simulink model "AOO"  (R2020a)
settings: Solver=FixedStepAuto  StartTime=0.0  StopTime=10.0  FixedStep=1e-3  RelTol=1e-3  EnableMultiTasking=on
undefined symbols (not defined in the file): D10, D11, D12, D2, D4, D5, D7, D8, D9, PTA0, PTA2, PTB23, PTB9, PTC3, PTC4, PTD0, PTD2, PTD3
libraries: frdmk64flib x11
settings Model: ExtModeTrigDuration=5  Creator=Hasan  LastModifiedBy=Hasan
settings OptimizationCC: EnhancedBackFolding=on  PassReuseOutputArgsAs=Individual arguments  ZeroExternalMemoryAtStartup=off  ZeroInternalMemoryAtStartup=off  MaxStackSize=64  OptimizeBlockOrder=speed  DifferentSizesBufferReuse=on  OptimizationCustomize=off  EfficientTunableParamExpr=on
settings DebuggingCC: ParameterTunabilityLossMsg=error
settings HardwareCC: ProdBitPerPointer=32  ProdBitPerSizeT=32  ProdBitPerPtrDiffT=32  ProdLargestAtomicInteger=Long  ProdLargestAtomicFloat=Double  ProdWordSize=32  ProdHWDeviceType=ARM Compatible->ARM Cortex
settings SFSimCC: MATLABDynamicMemAlloc=off
settings RTWCC: SystemTargetFile=ert.tlc  HardwareBoard=NXP FRDM-K64F  TemplateMakefile=ert_default_tmf  Toolchain=GNU Tools for ARM Embedded Processors
settings CodeAppCC: ForceParamTrailComments=on  IgnoreCustomStorageClasses=off  OperatorAnnotations=on  SimulinkDataObjDesc=on  SFDataObjDesc=on  InsertBlockDesc=on

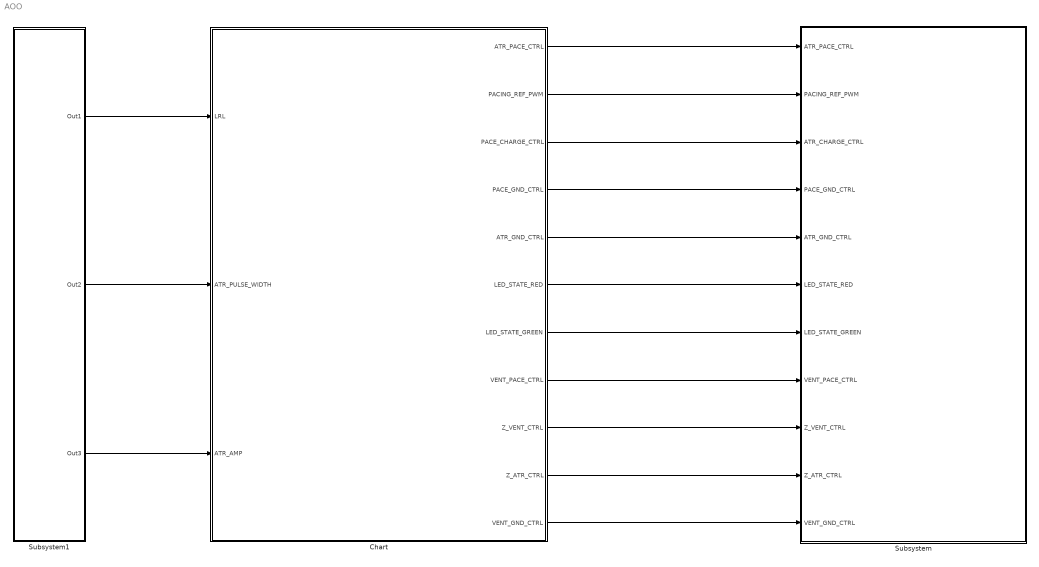
== system AOO ==
  Chart : Stateflow chart  TreatAsAtomicUnit=on
  Subsystem : Subsystem
  Subsystem1 : Subsystem
  wires:
  Chart/4(PACE_GND_CTRL) -> Subsystem/4(PACE_GND_CTRL)
  Chart/5(ATR_GND_CTRL) -> Subsystem/5(ATR_GND_CTRL)
  Chart/10(Z_ATR_CTRL) -> Subsystem/10(Z_ATR_CTRL)
  Chart/2(PACING_REF_PWM) -> Subsystem/2(PACING_REF_PWM)
  Chart/6(LED_STATE_RED) -> Subsystem/6(LED_STATE_RED)
  Chart/7(LED_STATE_GREEN) -> Subsystem/7(LED_STATE_GREEN)
  Chart/9(Z_VENT_CTRL) -> Subsystem/9(Z_VENT_CTRL)
  Chart/11(VENT_GND_CTRL) -> Subsystem/11(VENT_GND_CTRL)
  Chart/8(VENT_PACE_CTRL) -> Subsystem/8(VENT_PACE_CTRL)
  Chart/1(ATR_PACE_CTRL) -> Subsystem/1(ATR_PACE_CTRL)
  Chart/3(PACE_CHARGE_CTRL) -> Subsystem/3(ATR_CHARGE_CTRL)
  Subsystem1/1(Out1) -> Chart/1(LRL)
  Subsystem1/2(Out2) -> Chart/2(ATR_PULSE_WIDTH)
  Subsystem1/3(Out3) -> Chart/3(ATR_AMP)

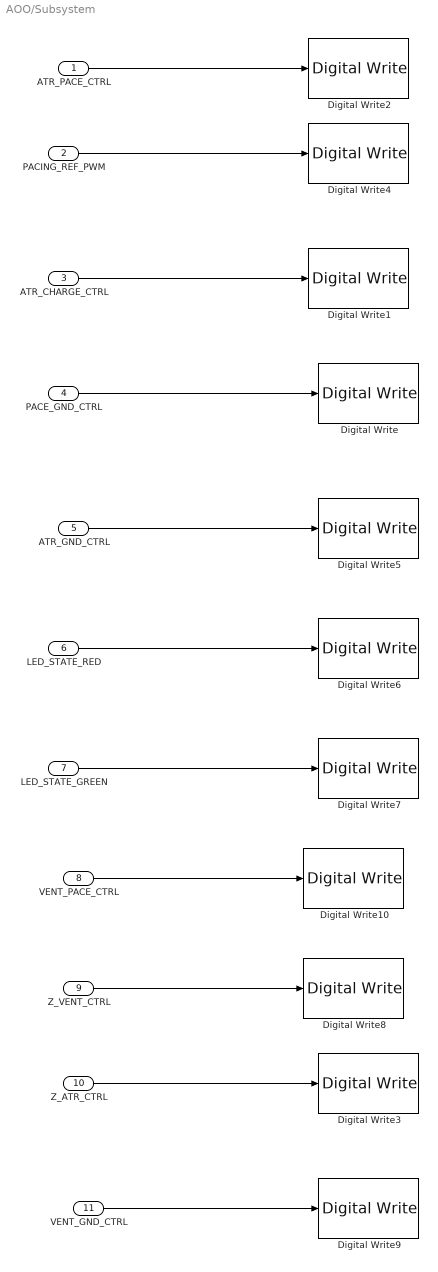
== system AOO/Subsystem ==
  ATR_PACE_CTRL : Inport
  PACING_REF_PWM : Inport  Port=2
  ATR_CHARGE_CTRL : Inport  Port=3
  PACE_GND_CTRL : Inport  Port=4
  ATR_GND_CTRL : Inport  Port=5
  LED_STATE_RED : Inport  Port=6
  LED_STATE_GREEN : Inport  Port=7
  VENT_PACE_CTRL : Inport  Port=8
  Z_VENT_CTRL : Inport  Port=9
  Z_ATR_CTRL : Inport  Port=10
  VENT_GND_CTRL : Inport  Port=11
  Digital Write : frdmk64flib/Digital Write  Whichpin=PTD0 (D10)
  Digital Write1 : frdmk64flib/Digital Write  Whichpin=PTB9 (D2)
  Digital Write10 : frdmk64flib/Digital Write  Whichpin=PTC4 (D9)
  Digital Write2 : frdmk64flib/Digital Write  Whichpin=PTA0 (D8)
  Digital Write3 : frdmk64flib/Digital Write  Whichpin=PTB23 (D4)
  Digital Write4 : frdmk64flib/Digital Write  Whichpin=PTA2 (D5)
  Digital Write5 : frdmk64flib/Digital Write  Whichpin=PTD2 (D11)
  Digital Write6 : frdmk64flib/Digital Write  Whichpin=RED_LED
  Digital Write7 : frdmk64flib/Digital Write  Whichpin=GREEN_LED
  Digital Write8 : frdmk64flib/Digital Write  Whichpin=PTC3 (D7)
  Digital Write9 : frdmk64flib/Digital Write  Whichpin=PTD3 (D12)
  wires:
  ATR_PACE_CTRL/1 -> Digital Write2/1
  PACING_REF_PWM/1 -> Digital Write4/1
  ATR_CHARGE_CTRL/1 -> Digital Write1/1
  VENT_GND_CTRL/1 -> Digital Write9/1
  Z_ATR_CTRL/1 -> Digital Write3/1
  Z_VENT_CTRL/1 -> Digital Write8/1
  VENT_PACE_CTRL/1 -> Digital Write10/1
  LED_STATE_GREEN/1 -> Digital Write7/1
  LED_STATE_RED/1 -> Digital Write6/1
  ATR_GND_CTRL/1 -> Digital Write5/1
  PACE_GND_CTRL/1 -> Digital Write/1

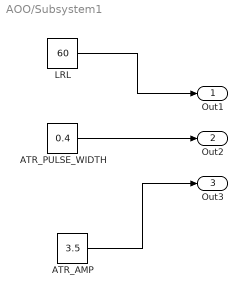
== system AOO/Subsystem1 ==
  ATR_AMP : Constant  Value=3.5  OutDataTypeStr=double
  ATR_PULSE_WIDTH : Constant  Value=0.4  OutDataTypeStr=double
  LRL : Constant  Value=60  OutDataTypeStr=double
  Out1 : Outport
  Out2 : Outport  Port=2
  Out3 : Outport  Port=3
  wires:
  ATR_AMP/1 -> Out3/1
  ATR_PULSE_WIDTH/1 -> Out2/1
  LRL/1 -> Out1/1

== stateflow chart AOO/Chart ==
  state AOO_INTERVAL_TIMER
    entry:
    ATR_PACE_CTRL = 0;
    PACE_CHARGE_CTRL = 1;
    PACING_REF_PWM = ATR_AMP;
    ATR_GND_CTRL = 1;
    PACE_GND_CTRL = 1;
    VENT_PACE_CTRL = 0;
    VENT_GND_CTRL = 0;
    Z_ATR_CTRL = 0;
    LED_STATE_RED=true;
    LED_STATE_GREEN=false;
  state AOO_PACE_DELIVERY
    entry:
    ATR_PACE_CTRL = 1;
    PACE_CHARGE_CTRL = 0;
    ATR_GND_CTRL = 0;
    PACE_GND_CTRL = 1;
    VENT_PACE_CTRL = 0;
    VENT_GND_CTRL = 0;
    Z_VENT_CTRL = 0;
    LED_STATE_RED=false;
    LED_STATE_GREEN=true;
  AOO_INTERVAL_TIMER -> AOO_PACE_DELIVERY : [after(60000/LRL-ATR_PULSE_WIDTH,msec)]
  AOO_PACE_DELIVERY -> AOO_INTERVAL_TIMER : [after(ATR_PULSE_WIDTH,msec)]
  (default) -> AOO_INTERVAL_TIMER
  data: ATR_PACE_CTRL output; PACING_REF_PWM output; PACE_CHARGE_CTRL output; PACE_GND_CTRL output; ATR_GND_CTRL output; LED_STATE_RED output; LED_STATE_GREEN output; VENT_PACE_CTRL output; Z_VENT_CTRL output; Z_ATR_CTRL output; VENT_GND_CTRL output; LRL input; ATR_PULSE_WIDTH input; ATR_AMP input
